simulink model "s_heli3dmpcdynamic (1)"  (R2024a)
settings: Solver=ode1  StartTime=0.0  StopTime=60  FixedStep=0.002  RelTol=1e-3  EnableMultiTasking=on
values from neighbouring files (symbols this model uses):
  CMD_RATE_LIMIT = 45.0 * pi / 180    (= 0.785398163397)    [lab_heli_3dmpc.m]    (also in setup_lab_heli_3d (1).m)
  K_AMP = 3    [lab_heli_3dmpc.m]    (also in setup_lab_heli_3d (1).m)
  kf = 9    [lab_heli_3dmpc.m]    (also in setup_lab_heli_3d (1).m = 15)
  VMAX_AMP = 24    [lab_heli_3dmpc.m]    (also in setup_lab_heli_3d (1).m)
  VMAX_DAC = 10    [lab_heli_3dmpc.m]    (also in setup_lab_heli_3d (1).m)
undefined symbols (not defined in the file or in its folder): A, Akf, B, Bkf, Ckf, D_cal, E_cal, Omu, Omx, Qkf, Rkf, Wu, Wx
libraries: simulink_extras x3
settings Model: ExtModeTrigDuration=5000  Creator=MLevis
settings SolverCC: AlgebraicLoopSolver=TrustRegion  PositivePriorityOrder=on
settings DataIOCC: LimitDataPoints=on  SaveFormat=Array  SignalLoggingSaveFormat=ModelDataLogs  ReturnWorkspaceOutputs=off
settings OptimizationCC: BooleanDataType=off  OptimizeBlockIOStorage=off  BufferReuse=off  ExpressionFolding=off  ExpressionDepthLimit=2147483647  LocalBlockOutputs=off  InitFltsAndDblsToZero=on  LifeSpan=inf
settings DebuggingCC: SaveWithParameterizedLinksMsg=none  UnderspecifiedInitializationDetection=Classic  MergeDetectMultiDrivingBlocksExec=none  SignalResolutionControl=TryResolveAllWithWarning  SolverPrmCheckMsg=warning  MultiTaskDSMMsg=warning  MultiTaskCondExecSysMsg=none  FcnCallInpInsideContextMsg=warning  UnconnectedInputMsg=warning  UnconnectedOutputMsg=warning  UnconnectedLineMsg=warning  StateNameClashWarn=warning  SFUnexpectedBacktrackingDiag=warning  SFNoUnconditionalDefaultTransitionDiag=warning  SFExecutionAtInitializationDiag=none  ArithmeticOperatorsInVariantConditions=warning
settings HardwareCC: ProdBitPerPointer=32  ProdBitPerSizeT=32  ProdBitPerPtrDiffT=32  ProdLargestAtomicFloat=None  ProdIntDivRoundTo=Undefined  ProdEndianess=Unspecified  ProdWordSize=32  ProdHWDeviceType=32-bit Generic
settings ModelReferenceCC: PropagateSignalLabelsOutOfModel=off
settings RTWCC: Description=QUARC Win32 Target  SystemTargetFile=quarc_windows.tlc  TemplateMakefile=quarc_default_tmf  GPUComputeCapability=3.5
settings CodeAppCC: StateflowObjectComments=on
settings STFCustomTargetCC: TargetFcnLib=ansi_tfl_tmw.mat  TargetPreCompLibLocation=C:\DOCUME~1\ALLUSE~1\APPLIC~1\QUARC\lib\2007a\windows\release  TargetLangStandard=C89/C90 (ANSI)  CPPClassGenCompliant=on  UseToolchainInfoCompliant=off  SystemTargetFile=quarc_windows.tlc
settings GRTTargetCC: TargetFcnLib=ansi_tfl_tmw.mat  TargetPreCompLibLocation=C:\DOCUME~1\ALLUSE~1\APPLIC~1\QUARC\lib\2007a\windows\release  TargetLangStandard=C89/C90 (ANSI)  ParMdlRefBuildCompliant=off  CompOptLevelCompliant=off  ConcurrentExecutionCompliant=off  CombineOutputUpdateFcns=off  MatFileLogging=off  GRTInterface=on  UseToolchainInfoCompliant=off  ExtMode=on  ExtModeMexFile=quarc_comm
settings ConfigComp: CovMetricSettings=dw  CovSaveCumulativeToWorkspaceVar=on  CovSaveSingleToWorkspaceVar=on

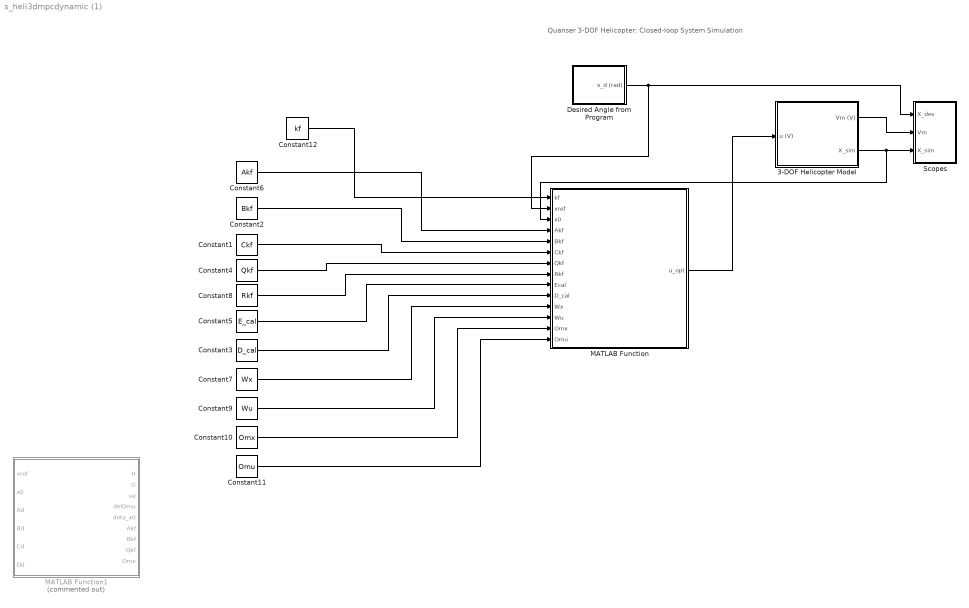
== system s_heli3dmpcdynamic (1) ==
  note: Quanser 3-DOF Helicopter:
      | Closed-loop System Simulation
  3-DOF Helicopter Model : Subsystem
  Constant1 : Constant  Value=Ckf
  Constant10 : Constant  Value=Omx
  Constant11 : Constant  Value=Omu
  Constant12 : Constant  Value=kf
  Constant2 : Constant  Value=Bkf
  Constant3 : Constant  Value=D_cal
  Constant4 : Constant  Value=Qkf
  Constant5 : Constant  Value=E_cal
  Constant6 : Constant  Value=Akf
  Constant7 : Constant  Value=Wx
  Constant8 : Constant  Value=Rkf
  Constant9 : Constant  Value=Wu
  Desired Angle from Program : Subsystem
  MATLAB Function : MATLAB Function  TreatAsAtomicUnit=on
  MATLAB Function1 : MATLAB Function  Commented=on  TreatAsAtomicUnit=on
  Scopes : Subsystem
  wires:
  Desired Angle from Program/1(x_d (rad)) -> Scopes/1(X_des), MATLAB Function/2(xref)
  MATLAB Function/1(u_opt) -> 3-DOF Helicopter Model/1(u (V))
  3-DOF Helicopter Model/2(X_sim) -> MATLAB Function/3(x0), Scopes/3(X_sim)
  3-DOF Helicopter Model/1(Vm (V)) -> Scopes/2(Vm)
  Constant7/1 -> MATLAB Function/11(Wx)
  Constant9/1 -> MATLAB Function/12(Wu)
  Constant10/1 -> MATLAB Function/13(Omx)
  Constant11/1 -> MATLAB Function/14(Omu)
  Constant6/1 -> MATLAB Function/4(Akf)
  Constant2/1 -> MATLAB Function/5(Bkf)
  Constant1/1 -> MATLAB Function/6(Ckf)
  Constant4/1 -> MATLAB Function/7(Qkf)
  Constant8/1 -> MATLAB Function/8(Rkf)
  Constant5/1 -> MATLAB Function/9(Ecal)
  Constant3/1 -> MATLAB Function/10(D_cal)
  Constant12/1 -> MATLAB Function/1(kf)

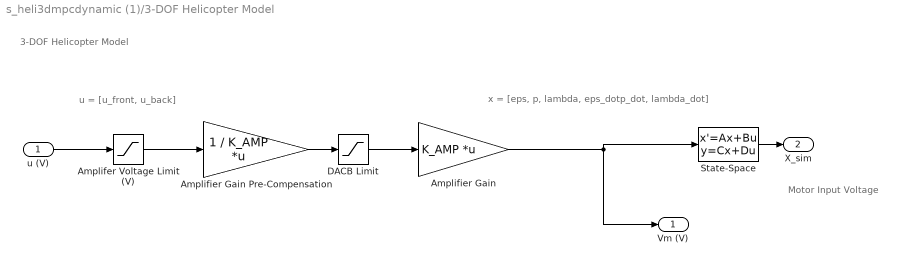
== system s_heli3dmpcdynamic (1)/3-DOF Helicopter Model ==
  note: x = [eps, p, lambda, eps_dotp_dot, lambda_dot]
  note: u = [u_front, u_back]
  note: Motor Input Voltage
  note: 3-DOF Helicopter Model
  u (V) : Inport
  Amplifer Voltage Limit (V) : Saturate  UpperLimit=VMAX_AMP  LowerLimit=-VMAX_AMP
  Amplifier Gain : Gain  Gain=K_AMP  Multiplication=Matrix(K*u)  SaturateOnIntegerOverflow=on  OutDataTypeStr=Inherit: Same as input  ParamDataTypeStr=Inherit: Same as input
  Amplifier Gain Pre-Compensation : Gain  Gain=1 / K_AMP  Multiplication=Matrix(K*u)  SaturateOnIntegerOverflow=on  OutDataTypeStr=Inherit: Same as input  ParamDataTypeStr=Inherit: Same as input
  DACB Limit : Saturate  UpperLimit=VMAX_DAC  LowerLimit=-VMAX_DAC
  State-Space : StateSpace  A=A  B=B  C=eye(6,6)  D=zeros(6,2)  InitialCondition=0
  Vm (V) : Outport
  X_sim : Outport  Port=2
  wires:
  u (V)/1 -> Amplifer Voltage Limit (V)/1
  State-Space/1 -> X_sim/1
  Amplifer Voltage Limit (V)/1 -> Amplifier Gain Pre-Compensation/1
  Amplifier Gain Pre-Compensation/1 -> DACB Limit/1
  DACB Limit/1 -> Amplifier Gain/1
  Amplifier Gain/1 -> State-Space/1, Vm (V)/1

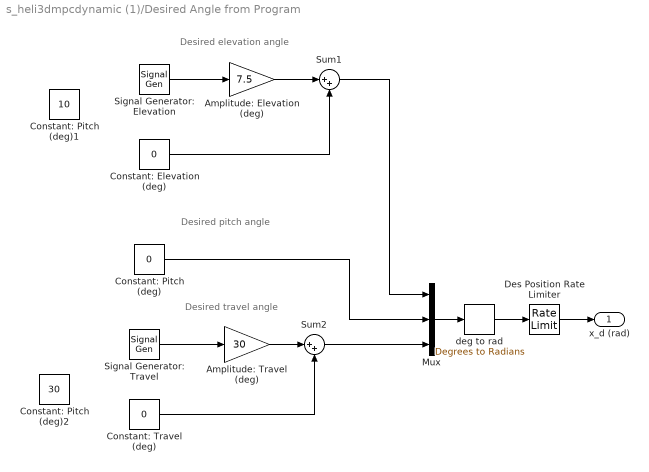
== system s_heli3dmpcdynamic (1)/Desired Angle from Program ==
  note: Desired elevation angle
  note: Desired travel angle
  note: Desired pitch angle
  Amplitude: Elevation (deg) : Gain  Gain=7.5
  Amplitude: Travel (deg) : Gain  Gain=30
  Constant: Elevation (deg) : Constant  Value=0
  Constant: Pitch (deg) : Constant  Value=0
  Constant: Pitch (deg)1 : Constant  Value=10
  Constant: Pitch (deg)2 : Constant  Value=30
  Constant: Travel (deg) : Constant  Value=0
  Des Position Rate Limiter : RateLimiter  RisingSlewLimit=CMD_RATE_LIMIT  FallingSlewLimit=-CMD_RATE_LIMIT  SampleTimeMode=inherited
  Mux : Mux  Inputs=3
  Signal Generator: Elevation : SignalGenerator  WaveForm=square  Frequency=0.04
  Signal Generator: Travel : SignalGenerator  WaveForm=square  Frequency=0.03
  Sum1 : Sum  Inputs=|++
  Sum2 : Sum  Inputs=|++
  deg to rad : simulink_extras/Transformations/Degrees to Radians
  x_d (rad) : Outport
  wires:
  Mux/1 -> deg to rad/1
  Constant: Elevation (deg)/1 -> Sum1/2
  Amplitude: Elevation (deg)/1 -> Sum1/1
  Signal Generator: Elevation/1 -> Amplitude: Elevation (deg)/1
  Constant: Travel (deg)/1 -> Sum2/2
  Amplitude: Travel (deg)/1 -> Sum2/1
  Signal Generator: Travel/1 -> Amplitude: Travel (deg)/1
  deg to rad/1 -> Des Position Rate Limiter/1
  Constant: Pitch (deg)/1 -> Mux/2
  Des Position Rate Limiter/1 -> x_d (rad)/1
  Sum1/1 -> Mux/1
  Sum2/1 -> Mux/3

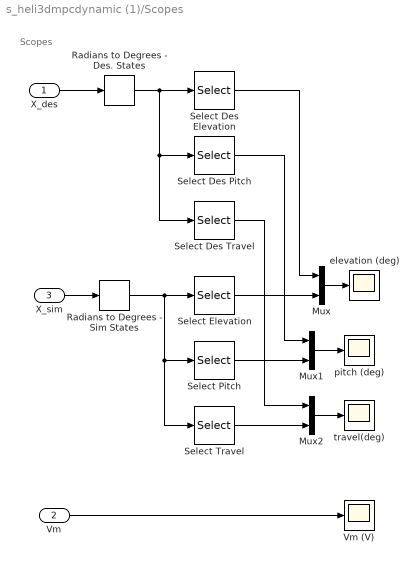
== system s_heli3dmpcdynamic (1)/Scopes ==
  note: Scopes
  X_des : Inport
  Vm : Inport  Port=2
  X_sim : Inport  Port=3
  Mux : Mux  Inputs=2
  Mux1 : Mux  Inputs=2
  Mux2 : Mux  Inputs=2
  Radians to Degrees - Des. States : simulink_extras/Transformations/Radians to Degrees
  Radians to Degrees - Sim States : simulink_extras/Transformations/Radians to Degrees
  Select Des Elevation : Selector  InputPortWidth=3  IndexOptions=Index vector (dialog)  Indices=1  OutputSizes=1
  Select Des Pitch : Selector  InputPortWidth=3  IndexOptions=Index vector (dialog)  Indices=2  OutputSizes=1
  Select Des Travel : Selector  InputPortWidth=3  IndexOptions=Index vector (dialog)  Indices=3  OutputSizes=1
  Select Elevation : Selector  InputPortWidth=6  IndexOptions=Index vector (dialog)  Indices=1  OutputSizes=1
  Select Pitch : Selector  InputPortWidth=6  IndexOptions=Index vector (dialog)  Indices=2  OutputSizes=1
  Select Travel : Selector  InputPortWidth=6  IndexOptions=Index vector (dialog)  Indices=3  OutputSizes=1
  Vm (V) : Scope
  elevation (deg) : Scope
  pitch (deg) : Scope
  travel(deg) : Scope
  wires:
  X_des/1 -> Radians to Degrees - Des. States/1
  X_sim/1 -> Radians to Degrees - Sim States/1
  Mux/1 -> elevation (deg)/1
  Mux1/1 -> pitch (deg)/1
  Vm/1 -> Vm (V)/1
  Radians to Degrees - Sim States/1 -> Select Elevation/1, Select Pitch/1, Select Travel/1
  Mux2/1 -> travel(deg)/1
  Select Elevation/1 -> Mux/2
  Select Pitch/1 -> Mux1/2
  Select Travel/1 -> Mux2/2
  Radians to Degrees - Des. States/1 -> Select Des Elevation/1, Select Des Pitch/1, Select Des Travel/1
  Select Des Elevation/1 -> Mux/1
  Select Des Pitch/1 -> Mux1/1
  Select Des Travel/1 -> Mux2/1

== matlab function s_heli3dmpcdynamic (1)/MATLAB Function1 ==
  data: xref input; H output; x0 input; Ad input; Bd input; Cd input; Dd input; G output; ue output; delOmu output; deta_x0 output; Akf output; Bkf output; Qkf output; Omx output
function [H, G, ue, delOmu, deta_x0,Akf, Bkf, Qkf, Omx] = mpc_controller(xref, x0, Ad, Bd, Cd, Dd)


%Ts = 0.1;
%sys_cont = ss(A, B, C, D);
%sys_disc = c2d(sys_cont,Ts, 'zoh');
%Ad = sys_disc.A;
%Bd = sys_disc.B;
%Cd = sys_disc.C;
%Dd = sys_disc.D;

display('Ad_total',[num2str(size(Ad))]);
display('xref',[num2str(size(xref))]);

%initial state condition
%x0 = [0;0;0;0;0;0];

% state and controller input constraints
uf_min = -24;
uf_max = 24;

ub_min = -24;
ub_max = 24;

elevation_min = deg2rad(-60); % min constraint of x1
elevation_max = deg2rad(60); %
pitch_min = deg2rad(-60);
pitch_max = deg2rad(60);
travel_min = deg2rad(-360);
travel_max = deg2rad(360);

%mpc controller 
kf = 4;              % prediction horizon

q1 = 10;            % penalize the elevation angle 
q2 = 1;             % penalize the pitch angle
q3 = 5;             % penalize the travel angle
q4 = 4;             % penalize the rate of change of the elevation angle
q5 = 6;             % penalize the rate of change of the pitch angle
q6 = 10;            % penalize the rate of change of the travel angle

r1 = 10;            % penalize the power of the front motor 
r2 = 5;             % penalize the power of the back motor

Q = diag([q1 q2 q3 q4 q5 q6]); % Weighting matrix for the states
R = diag([r1 r2]);             % Weighting matrix for the inputs


% State and Input Constraints
% state constraints

wx = [
    1 0 0 0 0 0;    % constrain epsilon 
    1 0 0 0 0 0;   % constrain -epsilon
    0 1 0 0 0 0;    % constrain rho
    0 1 0 0 0 0;   % constrain -rho
    0 0 1 0 0 0;    % constrain lambda
    0 0 1 0 0 0;   % constrain -lambda
];

omx =  [elevation_max;elevation_min;pitch_max;pitch_min;travel_max;travel_min];
% input constraints
wu = [1 0;
       1 0;
        0 1; 
        0 1];

omu = [uf_max;uf_min;ub_max;ub_min];
omxf = omx;
wxf = wx;

S = Q;


% Calculate the new equilibrium points
[nx, nu] = size(Bd);
[ny, ~] = size(Cd);

% Calculate the new equilibrium points
Ad_total = [Ad - eye(nx) Bd; Cd zeros(ny, nu)];
rhs = [zeros(nx, 1);xref];


xe_ue = Ad_total \ rhs;
xe = xe_ue(1:nx);
ue = xe_ue(nx+1:end);

% shitf states and inputs

del_omu = omu - wu*ue;
delta_x0 = x0 - xe;
delta_xref = xref - Cd*xe;


% condensed matrix computation
[Akf, Bkf] = Compute_Akf_Bkf(kf,Ad,Bd);
[Qkf, Rkf] = Compute_Qkf_Rkf(kf, Q, S, R);
[Wx, Omx, Wu, delOmu] = Compute_Wx_Omx_Wu_Omu(kf,wx,wxf,wu,omx,omxf,del_omu);

H = 2*(Rkf + Bkf'*Qkf*Bkf);    % define H for the quadratic program
G = [Wx*Bkf;
     Wu    ];                   % define G for the quadratic program
end

function [Akf, Bkf] = Compute_Akf_Bkf(kf, Ad, Bd)
[n, m] = size(Bd);   % number of states and inputs

Akf = zeros(n*(kf+1),n); % first block entry of Akf
Bkf = zeros(n*(kf+1), m*kf); %first block line of Bkf

Akf(1:n, 1:n) = eye(n);  % first block of kf


for i = 1:kf
  Akf(i*n+1:(i+1)*n, 1:n) = Ad^i;
  Bkfl = Ad^(i-1)*Bd;
  
  for l = 2:i
        Bkfl = [Bkfl, Ad^(i-l)*Bd];
  end
  
  Bkfl = [Bkfl, zeros(n,m*(kf-i))];
  Bkf(i*n+1:(i+1)*n,:) = Bkfl;

    end 
end


function [Wx, Omx, Wu, Omu] = Compute_Wx_Omx_Wu_Omu(kf,wx,wxf,wu,omx,omxf,omu)

[nw, nx] = size(wx);
[nu, mu] = size(wu);


Wx = zeros(nw*(kf+1),nx*(kf+1));
Omx = zeros(nw*(kf+1),1);
Wu =  zeros(nu*kf,mu*kf);
Omu = zeros(nu*kf,1);

for i = 1:kf

    Wx((i-1)*nw+1:i*nw,(i-1)*nx+1:i*nx) = wx;
    Omx((i-1)*nw+1:i*nw) = omx;

    Wu((i-1)*nu+1:i*nu,(i-1)*mu+1:i*mu) = wu;
    Omu((i-1)*nu+1:i*nu) = omu;
end

Wx(kf*nw+1:(kf+1)*nw, kf*nx+1:(kf+1)*nx) = wxf;
Omx(kf*nw+1:(kf+1)*nw) = omxf;

%Ue = repmat(ue, kf, 1);

%delOmu = Omu - Wu*Ue;

end

function [Qkf, Rkf] = Compute_Qkf_Rkf(kf, Q, S, R)

[nq, mq] = size(Q);
[nr, mr] = size(R);

Qkf = zeros(nq*(kf+1) , mq*(kf+1));
Rkf = zeros(nr*kf,mr*kf);


Qkf(1:nq,1:mq) = Q;
Rkf(1:nr, 1:mr) = R;

for i = 1:kf-1

    Qkf(i*nq+1:(i+1)*nq, i*mq+1:(i+1)*mq) = Q;

    Rkf(i*nr+1:(i+1)*nr,i*mr+1:(i+1)*mr) = R;
end
Qkf(kf*nq+1:(kf+1)*nq, kf*mq+1:(kf+1)*mq) = S;

end



%function [Wx, Omx, Wu, Omu] = Compute_Wx_Omx_Wu_Omu(kf,wx,wxf,wu,omx,omxf,omu, ue)
%Wu = wu;    % add first element to condensed W_u
%Omu = omu;  % add first element to condensed Omega_u

%Wx = wx;    % add first element to condensed W_x
%Omx = omx;  % add first element to condensed Omega_x

%for i = 0:kf-1 
 %   if i == kf-1
  %      Wx = blkdiag(Wu,wu);   % add last element to condesed W_x for the terminal state
   %     Omx = [Omx;omxf];      % add last element to condensed Omega_x for the terminal state
   % else
    %    Wu = blkdiag(Wu,wu); % add element to condesed W_u
     %   Omu = [Omu;omu];     % add element to condensed Omega_u

      %  Wx = blkdiag(Wx, wx);    % add element to condensed W_x
       % Omx = [Omx;omx];        % add element to condensed Omega_x
    %end

%end

% Modify Omu based on ue
%delOmu = Omu - Wu*ue;

%end



%function [Akf, Bkf] = Compute_Akf_Bkf(kf, Ad, Bd)
%[n, m] = size(Bd);   % number of states and inputs

%Akf = eye(n); % first block entry of Akf
%Bkf = zeros(n, m*kf); %first block line of Bkf

%for i = 1:kf
 %  Akf = [Akf;Ad^i]; % add always the new block to the power of i until kf
  % Bkfl = Ad^(i-1)*Bd; % this would be one line in the matrix of Bkf
%   for l = 2:i
%       Bkfl = [Bkfl, Ad^(i-l)*Bd]; % add the block entrys like defined in the lecture
%   end
 %  Bkfl = [Bkfl, zeros(n,m*(kf-i))];  % fill the rest of the blocks with zeros
%   Bkf = [Bkf;Bkfl];    % add the line to Bkf
%end
%end

%function Compute_Qkf_Rkf(kf, Q, S, R)

%Rkf = R; % add first element to Rkf
%Qkf = Q; % add first element to Qkf

%for i = 0:kf-1
 %   if i == kf-1
  %      Qkf =  blkdiag(Qkf, S); % add last element to Qkf for the terminal state
   %else 
    %    Rkf = blkdiag(Rkf,R);   % add element to Rkf
     %   Qkf = blkdiag(Qkf,Q);   % add elemnt to Qkf
  % end
%end
%end

== matlab function s_heli3dmpcdynamic (1)/MATLAB Function ==
  settings: updateMethod=DISCRETE
  data: kf input; xref input; u_opt output; x0 input; Akf input; Bkf input; Ckf input; Qkf input; Rkf input; Ecal input; D_cal input; Wx input; Wu input; Omx input; Omu input
function u_opt = mpcdynamic_controller(kf, xref, x0, Akf, Bkf,Ckf, Qkf, Rkf, Ecal, D_cal, Wx, Wu, Omx, Omu)
coder.extrinsic('quadprog');

persistent u_old

if isempty(u_old)
    u_old = zeros(2,1);
    u_opt = zeros(2,1);

end
xrefnew = [xref;1;1;1];   %change here the values therefore for the zeros and also for the gains for this three other states
Re = repmat(xrefnew, kf+1,1);


H = 2 * (Bkf' * Qkf * Bkf + (eye(length(D_cal)) - D_cal)' * Rkf * (eye(length(D_cal)) - D_cal));    % define H for the quadratic program
f = 2*(x0'*Akf'*Ckf'*Qkf*Ckf*Bkf - Re'*Qkf*Ckf*Bkf - u_old'*Ecal'*Rkf*(eye(length(D_cal)) - D_cal))';

G = [Wx*Bkf;
     Wu    ];                   % define G for the quadratic program

e = [Omx-Wx*Akf*x0;
    Omu         ];                % define e for the quadratic program


options = optimoptions('quadprog', 'Algorithm','active-set', 'Display','off');

%z0 = repmat(ue, kf,1);
z0 = zeros(size(f));

%z_opt = coder.nullcopy(zeros(nu*kf,1));

%z_opt = quadprog(H,f,G,e);

[z_opt, fval, exitflag, output] = quadprog(H,f,G,e, [],[],[],[],z0, options);  % solving of the optimization problem with constraints
% 
% if exitflag <= 0
%     warning('No feasible solution found. Quadprog exitflag: %d', exitflag);
%     disp(output.message);
%     u_opt = u_old; % Rückfall auf die vorherige Lösung
%     return;
% end


u_opt = z_opt(1:2);
u_old = u_opt;


end
